simulink model "CRCL"  (R2020b)
settings: Solver=FixedStepDiscrete  StartTime=0.0  StopTime=inf  FixedStep=0.01  RelTol=1e-3  EnableMultiTasking=on
values from neighbouring files (symbols this model uses):
  calibrationDelayTime_s = 2.0    [CRCL_Dictionary.sldd]
  collisionAngleThreshold_deg = 40.0    [CRCL_Dictionary.sldd]
  collisionVarianceThreshold_g2 = 8.0    [CRCL_Dictionary.sldd]
  cpMaxAbortTime_s = 30.0    [CRCL_Dictionary.sldd]
  cpMaxTipOverAngle_deg = 35.0    [CRCL_Dictionary.sldd]
  cpMinEstDistance_m = 50.0    [CRCL_Dictionary.sldd]
  cpMinEstDistanceGnssBased_m = 200.0    [CRCL_Dictionary.sldd]
  cpMinRiddenTime_s = 15.0    [CRCL_Dictionary.sldd]
  cpMinSpeedRiding_kmh = 10.0    [CRCL_Dictionary.sldd]
  cpNumCrankRevolutionThreshold = 5.0    [CRCL_Dictionary.sldd]
  cpSpeedCond2PositiveSpeedChangeTime_s = 5.0    [CRCL_Dictionary.sldd]
  cpSpeedDerivativeThreshold_kmhs = 0.005    [CRCL_Dictionary.sldd]
  cpTimeOutSpeedCond2_s = 15.0    [CRCL_Dictionary.sldd]
  groundHitEnergyThresholdStanding_g2s2 = 0.02    [CRCL_Dictionary.sldd]
  groundHitTipOverAngleThreshold_deg = 40.0    [CRCL_Dictionary.sldd]
  longAccCompForEulerEstFlag = 0.0    [CRCL_Dictionary.sldd]
  minEnergyStrongHit_g2s2 = 0.1    [CRCL_Dictionary.sldd]
  noMotionAccVarianceThresholdSD_g2 = 0.001    [CRCL_Dictionary.sldd]
  ride1minSpeedSlow_kmh = 4.0    [CRCL_Dictionary.sldd]
  ride2minSpeed_kmh = 8.0    [CRCL_Dictionary.sldd]
  rroMaxSpeed_kmh = 5.0    [CRCL_Dictionary.sldd]
  rroMinGyrX_degs = 20.0    [CRCL_Dictionary.sldd]
  rroMonotonyThreshold_degs = -1.0    [CRCL_Dictionary.sldd]
  rroRollIntegrationAngleThreshold_degs = 20.0    [CRCL_Dictionary.sldd]
  rroUniContinuityThreshold_degs = 15.0    [CRCL_Dictionary.sldd]
  scaleFactorVarianceStrongHit = 2.0    [CRCL_Dictionary.sldd]
  sdoMaxAccVarFreeFall_g2 = 0.06    [CRCL_Dictionary.sldd]
  sdoMaxTipOverAngle_deg = 20.0    [CRCL_Dictionary.sldd]
  sdoMinAccVar_g2 = 8.0    [CRCL_Dictionary.sldd]
  sdoMinGyrXYNorm_degs = 720.0    [CRCL_Dictionary.sldd]
  sdoMinGyrXYNormFreeFall_degs = 100.0    [CRCL_Dictionary.sldd]
  sdoMinOrientationChange_deg = 120.0    [CRCL_Dictionary.sldd]
  sdoScaleFactorOrientationChange = 3.0    [CRCL_Dictionary.sldd]
  stepTime_s = 0.01    [CRCL_Dictionary.sldd]
  strongHitSafetyFactor = 2.5    [CRCL_Dictionary.sldd]
  tipOverAccZFiltTreshold_g = 0.7    [CRCL_Dictionary.sldd]
  tipOverAngleThreshold_deg = 50.0    [CRCL_Dictionary.sldd]
  tipOverMinAccZFiltNoseOver_g = 0.3    [CRCL_Dictionary.sldd]
  tipOverRollPitchRelationNoseOver = 1.5    [CRCL_Dictionary.sldd]
undefined symbols (not defined in the file or in its folder): magnitude
libraries: simulink x17
(part 6 of 8)

== matlab function CRCL/MATLAB Function1 ==
  data: probRide1 input; p_noCrash output; probRide2 input; probSoftColl input; probColl input; probStrongColl input; probTipOver input; probNoseOver input; probGroundHit input; probRRO input; probSDO input; probHubConnection input; systemConfig input; p_crash output; crashClass output; outputCrashClass output; p_maxCrashClass output; tipOverAngleFused_deg input; outputGeneralCrashClass output; p_generalCrashClass output; cobiHubSetup input; p_cc1x output; p_cc3x output; secondCalibDoneDelayed input
function [p_noCrash, p_crash, crashClass, outputCrashClass, ...
    p_maxCrashClass, outputGeneralCrashClass, ...
    p_generalCrashClass, p_cc1x, p_cc3x] = crashProbabilityFusion(probRide1, probRide2, probSoftColl, ...
    probColl, probStrongColl, probTipOver, probNoseOver, probGroundHit, ...
    probRRO, probSDO, probHubConnection, systemConfig, ...
    tipOverAngleFused_deg, cobiHubSetup, secondCalibDoneDelayed)

persistent lastCrashClass probRide1Freeze ...
    probRide2Freeze rideFeatureFreeze lastCrashClassRanking ...
    crashClassHighestRanking generalCrashClassHighestRanking ...
    generalCrashClassProb

if isempty(lastCrashClass)
    lastCrashClass = single(0);
    probRide1Freeze = single(0);
    probRide2Freeze = single(0);
    rideFeatureFreeze = int16(0);
    lastCrashClassRanking = single(0);
    crashClassHighestRanking = int16(0);
    generalCrashClassHighestRanking = int16(0);
    generalCrashClassProb = single(0);
end

%ride feature freeze 
if (tipOverAngleFused_deg >= 50 || probGroundHit >= 0.5 || ...
        probColl >= 0.5) && rideFeatureFreeze == 0 && secondCalibDoneDelayed == 1
    probRide1Freeze = probRide1;
    probRide2Freeze = probRide2;
    rideFeatureFreeze = int16(1);
%reset frozen feature states and crash classes + probs
elseif  tipOverAngleFused_deg < 50 && probGroundHit < 0.5 && ...
        probColl < 0.5 && probTipOver < 0.5 && probSDO < 0.5 && ...
        ~(probHubConnection < 0.5 && systemConfig == 2) && rideFeatureFreeze == 1
    probRide1Freeze = probRide1;
    probRide2Freeze = probRide2;
    rideFeatureFreeze = int16(0);
    lastCrashClassRanking = single(0);
    crashClassHighestRanking = int16(0);
    generalCrashClassHighestRanking = int16(0);
    generalCrashClassProb = single(0);
elseif rideFeatureFreeze == 0
     probRide1Freeze = probRide1;
     probRide2Freeze = probRide2;
end
    
%% probabilistic tree

%% ride0
if probRide1Freeze < 0.3
    p_0 = 1 - probRide1Freeze;

    %collision node
    p_00 = p_0 * (1 - probSoftColl);                                    % -> no Collision
    p_01 = p_0 * probSoftColl * (1 - probColl) ;                        % -> soft Collsion
    p_02 = p_0 * probSoftColl * probColl * (1 - probStrongColl);        % -> Collision
    p_03 = p_0 * probSoftColl * probColl * probStrongColl;              % -> Strong Collision

    % tipover
    p_000 = p_00 * (1 - probTipOver);                                   %no TipOver
    p_001 = p_00 * probTipOver * (1 - probNoseOver);                    %RollOver
    p_002 = p_00 * probTipOver * probNoseOver;                          %NoseOver

    p_010 = p_01 * (1 - probTipOver);
    p_011 = p_01 * probTipOver * (1 - probNoseOver);
    p_012 = p_01 * probTipOver * probNoseOver;

    p_020 = p_02 * (1 - probTipOver);
    p_021 = p_02 * probTipOver * (1 - probNoseOver);
    p_022 = p_02 * probTipOver * probNoseOver;

    p_030 = p_03 * (1 - probTipOver);
    p_031 = p_03 * probTipOver * (1 - probNoseOver);
    p_032 = p_03 * probTipOver * probNoseOver;

    % ground hit node
    %not riding, no Collision
    p_0000 = p_000 * (1-probGroundHit);
    p_0001 = p_000 * probGroundHit;

    p_0010 = p_001 * (1-probGroundHit);
    p_0011 = p_001 * probGroundHit;

    p_0020 = p_002 * (1-probGroundHit);
    p_0021 = p_002 * probGroundHit;

    %not riding, softCollision
    p_0100 = p_010 * (1-probGroundHit);
    p_0101 = p_010 * probGroundHit;

    p_0110 = p_011 * (1-probGroundHit);
    p_0111 = p_011 * probGroundHit;

    p_0120 = p_012 * (1-probGroundHit);
    p_0121 = p_012 * probGroundHit;

    %not riding, Collision
    p_0200 = p_020 * (1-probGroundHit);
    p_0201 = p_020 * probGroundHit;

    p_0210 = p_021 * (1-probGroundHit);
    p_0211 = p_021 * probGroundHit;

    p_0220 = p_022 * (1-probGroundHit);
    p_0221 = p_022 * probGroundHit;

    %not riding, strong Collision
    p_0300 = p_030 * (1-probGroundHit);
    p_0301 = p_030 * probGroundHit;

    p_0310 = p_031 * (1-probGroundHit);
    p_0311 = p_031 * probGroundHit;

    p_0320 = p_032 * (1-probGroundHit);
    p_0321 = p_032 * probGroundHit;

    % special features
    % riderlessRollOver
    p_0011a = p_0011 * (1 - single(probRRO));
    p_0011b = p_0011 * single(probRRO);


    p_1000 = single(0);
    p_1001 = single(0);
    p_1010 = single(0);
    p_1011 = single(0);
    p_1020 = single(0);
    p_1021 = single(0);
    p_1200 = single(0);
    p_1201 = single(0);
    p_1210 = single(0);
    p_1211 = single(0);
    p_1220 = single(0);
    p_1221 = single(0);
    p_1300 = single(0);
    p_1301 = single(0);
    p_1310 = single(0);
    p_1311 = single(0);
    p_1320 = single(0);
    p_1321 = single(0);
    
    p_2000 = single(0);
    p_2001 = single(0);
    p_2010 = single(0);
    p_2011 = single(0);
    p_2020 = single(0);
    p_2021 = single(0);
    p_2200 = single(0);
    p_2201 = single(0);
    p_2210 = single(0);
    p_2211 = single(0);
    p_2220 = single(0);
    p_2221 = single(0);
    p_2300 = single(0);
    p_2301 = single(0);
    p_2310 = single(0);
    p_2311 = single(0);
    p_2320 = single(0);
    p_2321 = single(0);

else
    %% ride1
    p_1 = probRide1Freeze * (1-probRide2Freeze);

    %collision node
    p_10 = p_1 * (1 - probColl);                                        % -> no Collison
    p_12 = p_1 * probColl * (1 - probStrongColl);                       % -> Collision
    p_13 = p_1 * probColl * probStrongColl;                             % -> strongCollsion

    % tipover
    p_100 = p_10 * (1 - probTipOver);
    p_101 = p_10 * probTipOver * (1 - probNoseOver);
    p_102 = p_10 * probTipOver * probNoseOver;

    p_120 = p_12 * (1 - probTipOver);
    p_121 = p_12 * probTipOver * (1 - probNoseOver);
    p_122 = p_12 * probTipOver * probNoseOver;

    p_130 = p_13 * (1 - probTipOver);
    p_131 = p_13 * probTipOver * (1 - probNoseOver);
    p_132 = p_13 * probTipOver * probNoseOver;

    % ground hit node
    %riding 1, no Collision
    p_1000 = p_100 * (1-probGroundHit);
    p_1001 = p_100 * probGroundHit;

    p_1010 = p_101 * (1-probGroundHit);
    p_1011 = p_101 * probGroundHit;

    p_1020 = p_102 * (1-probGroundHit);
    p_1021 = p_102 * probGroundHit;

    %riding 1, Collision
    p_1200 = p_120 * (1-probGroundHit);
    p_1201 = p_120 * probGroundHit;

    p_1210 = p_121 * (1-probGroundHit);
    p_1211 = p_121 * probGroundHit;

    p_1220 = p_122 * (1-probGroundHit);
    p_1221 = p_122 * probGroundHit;

    %riding 1, strong Collision
    p_1300 = p_130 * (1-probGroundHit);
    p_1301 = p_130 * probGroundHit;

    p_1310 = p_131 * (1-probGroundHit);
    p_1311 = p_131 * probGroundHit;

    p_1320 = p_132 * (1-probGroundHit);
    p_1321 = p_132 * probGroundHit;

    %% ride2
    p_2 = probRide1Freeze * probRide2Freeze;

    %collision node
    p_20 = p_2 * (1 - probColl);                                        % -> no Collison
    p_22 = p_2 * probColl * (1 - probStrongColl);                       % -> Collision
    p_23 = p_2 * probColl * probStrongColl;                             % -> strongCollsion

    % tipover
    p_200 = p_20 * (1 - probTipOver);
    p_201 = p_20 * probTipOver * (1 - probNoseOver);
    p_202 = p_20 * probTipOver * probNoseOver;

    p_220 = p_22 * (1 - probTipOver);
    p_221 = p_22 * probTipOver * (1 - probNoseOver);
    p_222 = p_22 * probTipOver * probNoseOver;

    p_230 = p_23 * (1 - probTipOver);
    p_231 = p_23 * probTipOver * (1 - probNoseOver);
    p_232 = p_23 * probTipOver * probNoseOver;

    % ground hit node
    %riding 2, no Collision
    p_2000 = p_200 * (1-probGroundHit);
    p_2001 = p_200 * probGroundHit;

    p_2010 = p_201 * (1-probGroundHit);
    p_2011 = p_201 * probGroundHit;

    p_2020 = p_202 * (1-probGroundHit);
    p_2021 = p_202 * probGroundHit;

    %riding 2, Collision
    p_2200 = p_220 * (1-probGroundHit);
    p_2201 = p_220 * probGroundHit;

    p_2210 = p_221 * (1-probGroundHit);
    p_2211 = p_221 * probGroundHit;

    p_2220 = p_222 * (1-probGroundHit);
    p_2221 = p_222 * probGroundHit;

    %riding 2, strong Collision
    p_2300 = p_230 * (1-probGroundHit);
    p_2301 = p_230 * probGroundHit;

    p_2310 = p_231 * (1-probGroundHit);
    p_2311 = p_231 * probGroundHit;

    p_2320 = p_232 * (1-probGroundHit);
    p_2321 = p_232 * probGroundHit;
    
    p_0000 = single(0);
    p_0001 = single(0);
    p_0010 = single(0);
    %p_0011 = single(0);
    p_0020 = single(0);
    p_0021 = single(0);
    p_0100 = single(0);
    p_0101 = single(0);
    p_0110 = single(0);
    p_0111 = single(0);
    p_0120 = single(0);
    p_0121 = single(0);
    p_0200 = single(0);
    p_0201 = single(0);
    p_0210 = single(0);
    p_0211 = single(0);
    p_0220 = single(0);
    p_0221 = single(0);
    p_0300 = single(0);
    p_0301 = single(0);
    p_0310 = single(0);
    p_0311 = single(0);
    p_0320 = single(0);
    p_0321 = single(0);
    p_0011a = single(0);
    p_0011b = single(0);
end

%% crashClasses

%no crash
p_cc00 = p_0000 + p_0001 + p_0010 + p_0020 + p_0100 + p_0101 + p_0110 + ...
    p_0120 + p_0200 + p_0201 + p_1000 + p_1001 + p_1010 + p_1020 + ...
    p_1200 + p_1201 + p_2000 + p_2001 + p_2200 + p_2201;
p_cc70 = p_0011b;
p_maxCrashClass = p_cc00;

crashClass = int16(0);
if lastCrashClassRanking <= 5 && p_cc00 > 0.5
    lastCrashClassRanking = single(5);
    crashClassHighestRanking = crashClass;
    generalCrashClassHighestRanking = int16(0);
    generalCrashClassProb = p_cc00 + p_cc70;
end


if p_cc70 > p_maxCrashClass
    p_maxCrashClass = p_cc70;
    crashClass = int16(70);
    if lastCrashClassRanking <= 7 && p_cc70 > 0.5
        lastCrashClassRanking = single(7);
        crashClassHighestRanking = crashClass;
        generalCrashClassHighestRanking = int16(0);
        generalCrashClassProb = p_cc00 + p_cc70;
    end
end

% crashes
p_cc10 = p_1210 + p_1211 + p_2210 + p_2211;
p_cc11 = p_1300 + p_1301 + p_2300 + p_2301;
p_cc12 = p_1220 + p_1221 + p_2220 + p_2221;
p_cc15 = p_1310 + p_1311 + p_2310 + p_2311;
p_cc16 = p_1320 + p_1321 + p_2320 + p_2321;

p_cc1x = p_cc10 + p_cc11 + p_cc12 + p_cc15 + p_cc16;

if p_cc10 > p_maxCrashClass
    p_maxCrashClass = p_cc10;
    crashClass = int16(10);
    if lastCrashClassRanking <= 30 && p_cc10 > 0.5
        lastCrashClassRanking = single(30);
        crashClassHighestRanking = crashClass;
        generalCrashClassHighestRanking = int16(1);
        generalCrashClassProb = p_cc1x;
    end
end
if p_cc11 > p_maxCrashClass
    p_maxCrashClass = p_cc11;
    crashClass = int16(11);
    if lastCrashClassRanking <= 25 && p_cc11 > 0.5
        lastCrashClassRanking = single(25);
        crashClassHighestRanking = crashClass;
        generalCrashClassHighestRanking = int16(1);
        generalCrashClassProb = p_cc1x;
    end
end
if p_cc12 > p_maxCrashClass
    p_maxCrashClass = p_cc12;
    crashClass = int16(12);
    if lastCrashClassRanking <= 30 && p_cc12 > 0.5
        lastCrashClassRanking = single(30);
        crashClassHighestRanking = crashClass;
        generalCrashClassHighestRanking = int16(1);
        generalCrashClassProb = p_cc1x;
    end
end
if p_cc15 > p_maxCrashClass
    p_maxCrashClass = p_cc15;
    crashClass = int16(15);
    if lastCrashClassRanking <= 30 && p_cc15 > 0.5
        lastCrashClassRanking = single(30);
        crashClassHighestRanking = crashClass;
        generalCrashClassHighestRanking = int16(1);
        generalCrashClassProb = p_cc1x;
    end
end
if p_cc16 > p_maxCrashClass
    p_maxCrashClass = p_cc16;
    crashClass = int16(16);
    if lastCrashClassRanking <= 30 && p_cc16 > 0.5
        lastCrashClassRanking = single(30);
        crashClassHighestRanking = crashClass;
        generalCrashClassHighestRanking = int16(1);
        generalCrashClassProb = p_cc1x;
    end
end

p_cc20 = p_2010 + p_2011;
p_cc22 = p_2020 + p_2021;

p_cc2x = p_cc20 + p_cc22;

if p_cc20 > p_maxCrashClass
    p_maxCrashClass = p_cc20;
    crashClass = int16(20);
    if lastCrashClassRanking <= 20 && p_cc20 > 0.5
        lastCrashClassRanking = single(20);
        crashClassHighestRanking = crashClass;
        generalCrashClassHighestRanking = int16(2);
        generalCrashClassProb = p_cc2x;
    end
end
if p_cc22 > p_maxCrashClass
    p_maxCrashClass = p_cc22;
    crashClass = int16(22);
    if lastCrashClassRanking <= 20 && p_cc22 > 0.5
        lastCrashClassRanking = single(20);
        crashClassHighestRanking = crashClass;
        generalCrashClassHighestRanking = int16(2);
        generalCrashClassProb = p_cc2x;
    end
end

p_cc30 = p_1011;
p_cc32 = p_1021;
p_cc33 = p_0011a + p_0021;

p_cc3x = p_cc30 + p_cc32 + p_cc33;

if p_cc30 > p_maxCrashClass 
    p_maxCrashClass = p_cc30;
    crashClass = int16(30);
    if lastCrashClassRanking <= 25 && p_cc30 > 0.5
        lastCrashClassRanking = single(25);
        crashClassHighestRanking = crashClass;
        generalCrashClassHighestRanking = int16(3);
        generalCrashClassProb = p_cc3x;
    end
end
if p_cc32 > p_maxCrashClass
    p_maxCrashClass = p_cc32;
    crashClass = int16(32);
    if lastCrashClassRanking <= 25 && p_cc32 > 0.5
        lastCrashClassRanking = single(25);
        crashClassHighestRanking = crashClass;
        generalCrashClassHighestRanking = int16(3);
        generalCrashClassProb = p_cc3x;
    end
end
if p_cc33 > p_maxCrashClass
    p_maxCrashClass = p_cc33;
    crashClass = int16(33);
    if lastCrashClassRanking <= 15 && p_cc33 > 0.5
        lastCrashClassRanking = single(15);
        crashClassHighestRanking = crashClass;
        generalCrashClassHighestRanking = int16(3);
        generalCrashClassProb = p_cc3x;
    end
end


p_cc40 = p_0111 + p_0121;
p_cc41 = p_0300 + p_0301;
p_cc44 = p_0210 + p_0211 + p_0220 + p_0221;
p_cc45 = p_0310 + p_0311 + p_0320 + p_0321;
p_cc4x = p_cc41 + p_cc40 + p_cc44 + p_cc45;

if p_cc40 > p_maxCrashClass
    p_maxCrashClass = p_cc40;
    crashClass = int16(40);
    if lastCrashClassRanking <= 25 && p_cc40 > 0.5
        lastCrashClassRanking = single(25);
        crashClassHighestRanking = crashClass;
        generalCrashClassHighestRanking = int16(4);
        generalCrashClassProb = p_cc4x;
    end
end
if p_cc41 > p_maxCrashClass
    p_maxCrashClass = p_cc41;
    crashClass = int16(41);
    if lastCrashClassRanking <= 10 && p_cc41 > 0.5
        lastCrashClassRanking = single(10);
        crashClassHighestRanking = crashClass;
        generalCrashClassHighestRanking = int16(4);
        generalCrashClassProb = p_cc4x;
    end
end
if p_cc44 > p_maxCrashClass
    p_maxCrashClass = p_cc44;
    crashClass = int16(44);
    if lastCrashClassRanking <= 20 && p_cc44 > 0.5
        lastCrashClassRanking = single(20);
        crashClassHighestRanking = crashClass;
        generalCrashClassHighestRanking = int16(4);
        generalCrashClassProb = p_cc4x;
    end
end
if p_cc45 > p_maxCrashClass
    p_maxCrashClass = p_cc45;
    crashClass = int16(45);
    if lastCrashClassRanking <= 20 && p_cc45 > 0.5
        lastCrashClassRanking = single(20);
        crashClassHighestRanking = crashClass;
        generalCrashClassHighestRanking = int16(4);
        generalCrashClassProb = p_cc4x;
    end
end




%% output 
p_noCrash = p_cc00 + p_cc70;

p_crash = p_cc10 + p_cc11 + p_cc12 + p_cc15 + p_cc16 + p_cc20 + p_cc22 + ...
    p_cc30 + p_cc32 + p_cc33 + p_cc40 + p_cc41 + p_cc44 + p_cc45;

% cobi special cases
if systemConfig == 2 && probHubConnection == 0  && ... % lost hub
        cobiHubSetup ~= 1 && ...
        (probColl >= 0.5 || probGroundHit >= 0.5)
    lastCrashClassRanking = single(50);
    generalCrashClassHighestRanking = int16(8);
    generalCrashClassProb = single(1);
    if probRide1Freeze >= 0.5   %riding
        crashClass = int16(81);
        crashClassHighestRanking = crashClass;
        lastCrashClassRanking = single(55);
        %p_maxCrashClass = single(1);
    else                            % not riding
        crashClass = int16(80);
        crashClassHighestRanking = crashClass;
        lastCrashClassRanking = single(50);
        %p_maxCrashClass = single(1);    
    end
elseif systemConfig == 2 && probHubConnection == 1 && ...
        probSDO >= 0.9 % smartphone drop out cases
    p_crash = single(1);
    p_noCrash = single(0);
    generalCrashClassHighestRanking = int16(8);
    generalCrashClassProb = single(1);
    if lastCrashClassRanking < single(50)
        if probRide1Freeze >= 0.5   %riding
            crashClass = int16(83);
            crashClassHighestRanking = crashClass;
            lastCrashClassRanking = single(45);
            %p_maxCrashClass = single(1);
        else                        %not riding
            crashClass = int16(82);
            crashClassHighestRanking = crashClass;
            lastCrashClassRanking = single(40);
            %p_maxCrashClass = single(1);   
        end
    end
end

outputCrashClass = crashClassHighestRanking;
outputGeneralCrashClass = generalCrashClassHighestRanking;
p_generalCrashClass = generalCrashClassProb;

% if
%     outputCrashClass
% else
%     outputCrashClass
% end

end

== stateflow chart CRCL/CP_crashPlausiblizer ==
  state plausibilityChecker [parallel]
    settings: executionOrder=1
    state Idle_
      en:
      CP_fire = int16(0);
      CP_crashAborted = int16(0);
      CP_plausibleCrashClass =int16(0);
    state plausibleCrash
      en:
      CP_fire = int16(1);
      CP_plausibleCrashClass =CP_crashClassTmp;
      du:
      if CP_curCrashClass ~=0  && ...
      CP_crashClassTmp ~= CP_curCrashClass
      CP_crashClassTmp = CP_curCrashClass;
      CP_plausibleCrashClass =CP_crashClassTmp;
      end
    state CrashDetected
      du:
      if CP_curCrashClass ~=0  && ...
      CP_crashClassTmp ~= CP_curCrashClass
      CP_crashClassTmp = CP_curCrashClass;
      end
    state unplausibleCrash
      en:
      CP_crashAborted = int16(1);
    plausibleCrash -> Idle_ : [CP_crashFire == 0 && after(5,sec)]
    (default) -> Idle_
    Idle_ -> plausibilityChecker.CrashDetected : [CP_crashFire ==1]
        | {
        | CP_crashClassTmp = CP_curCrashClass;
        | }
    plausibilityChecker.CrashDetected -> plausibleCrash [order 1] : [CP_standFire || ...
        | CP_crashClass >= 80 || ...
        | CP_curSpeed_kmh < CP_minSpeedRiding_kmh || ...
        | after(CP_maxAbortTime_s,sec)]
        | %&& ...
        | %CP_speedCondFire == 0 && ...
        | %CP_cadenceCondFire == 0 && ...
        | %CP_speedCond2Fire == 0)]
    plausibilityChecker.CrashDetected -> unplausibleCrash [order 2] : [CP_speedCondFire == 2 || ...
        | CP_cadenceCondFire == 2 || ...
        | CP_speedCond2Fire == 2 || ...
        | CP_gnssSpeedCondFire == 2]
    unplausibleCrash -> Idle_ : [CP_crashFire == 0]
  state speedUprigthBikeConditionChecker [parallel]
    settings: executionOrder=2
    state waitState
    state SpeedConditionValid
      en:
      CP_speedCondFire = int16(1);
      CP_intDistance_m = CP_timeStep_s * CP_curSpeed_kmh/3.6;
      du:
      CP_intDistance_m  = CP_intDistance_m + CP_timeStep_s * CP_curSpeed_kmh/3.6;
    state Idle
      en:
      CP_speedCondFire = int16(0);
    state CrashDetected
      en:
      CP_speedCondFire = int16(0);
    state wait
    speedUprigthBikeConditionChecker.SpeedConditionValid -> speedUprigthBikeConditionChecker.waitState [order 1] : [after(CP_minRiddenTime_s,sec) && CP_intDistance_m >= CP_minEstDistance_m]
        | {
        | CP_speedCondFire = int16(2);
        | }
    speedUprigthBikeConditionChecker.waitState -> speedUprigthBikeConditionChecker.Idle : [after(1,sec)]
    speedUprigthBikeConditionChecker.Idle -> speedUprigthBikeConditionChecker.CrashDetected [commented out] : [CP_crashFire ==1]
    speedUprigthBikeConditionChecker.CrashDetected -> speedUprigthBikeConditionChecker.SpeedConditionValid [order 1] : %check if bicycle is upright and backwheel is rotating
        | [CP_curSpeed_kmh > CP_minSpeedRiding_kmh && ...
        | (CP_tipOverAngleFused_deg <= CP_maxTipOverAngle_deg && ...
        | CP_tipOverAngleAcc_deg <= CP_maxTipOverAngle_deg)]
    speedUprigthBikeConditionChecker.CrashDetected -> speedUprigthBikeConditionChecker.Idle [commented out] : [CP_crashFire ==0 && after(15,sec)]
    (default) -> speedUprigthBikeConditionChecker.Idle
    speedUprigthBikeConditionChecker.SpeedConditionValid -> speedUprigthBikeConditionChecker.CrashDetected [order 2] : [CP_curSpeed_kmh < CP_minSpeedRiding_kmh || ...
        | CP_tipOverAngleFused_deg > CP_maxTipOverAngle_deg || ...
        | CP_tipOverAngleAcc_deg > CP_maxTipOverAngle_deg]
    speedUprigthBikeConditionChecker.Idle -> speedUprigthBikeConditionChecker.CrashDetected [order 1] : [CP_crashFire ==1 && ...
        | CP_curSpeed_kmh >= CP_minSpeedRiding_kmh]
    speedUprigthBikeConditionChecker.CrashDetected -> speedUprigthBikeConditionChecker.wait [order 2] : [CP_curSpeed_kmh < CP_minSpeedRiding_kmh || after(CP_maxAbortTime_s,sec)]
    speedUprigthBikeConditionChecker.wait -> speedUprigthBikeConditionChecker.Idle : [CP_crashFire ==0]
    speedUprigthBikeConditionChecker.Idle -> speedUprigthBikeConditionChecker.wait [order 2] : [CP_crashFire ==1 && ...
        | CP_curSpeed_kmh < CP_minSpeedRiding_kmh]
  state cadenceConditionChecker [parallel]
    settings: executionOrder=3
    state waitState
    state Idle
      en:
      CP_cadenceCondFire = int16(0);
    state checkCadenceCondition
      en:
      CP_cadenceCondFire = int16(1);
      du:
      CP_crankRotation = CP_curCadence/60 * CP_timeStep_s + CP_crankRotation;
    state CrashDetected
      en:
      CP_cadenceCondFire = int16(0);
      CP_crankRotation = single(0);
    state waitState1
    state wait
      en:
      CP_cadenceCondFire = int16(0);
    cadenceConditionChecker.waitState -> cadenceConditionChecker.Idle : [after(1,sec)]
    checkCadenceCondition -> cadenceConditionChecker.waitState [order 2] : %cadence condition valid
        | [CP_crankRotation >= CP_numCrankRevolutionThreshold]
        | {
        | CP_cadenceCondFire = int16(2);
        | }
    cadenceConditionChecker.CrashDetected -> checkCadenceCondition [order 1] : %check if user applies valid cadence
        | [CP_curCadence >= 30 && CP_curCadence <= 150]
        | %(CP_tipOverAngleFused_deg <= 35 && ...
        | %CP_tipOverAngleAcc_deg <= 35)]
    cadenceConditionChecker.Idle -> cadenceConditionChecker.CrashDetected [order 1] : [CP_crashFire ==1 && ...
        | CP_curSpeed_kmh > CP_minSpeedRiding_kmh]
    (default) -> cadenceConditionChecker.Idle
    checkCadenceCondition -> waitState1 [order 1] : [CP_curCadence < 30 || ...
        | CP_curCadence > 150]
    cadenceConditionChecker.CrashDetected -> cadenceConditionChecker.Idle [commented out] : [CP_crashFire == 0 && after(25,sec)]
    waitState1 -> cadenceConditionChecker.CrashDetected [order 2] : [after(5,sec)]
    waitState1 -> checkCadenceCondition [order 1] : [CP_curCadence >= 30  && ...
        | CP_curCadence <= 150]
    cadenceConditionChecker.CrashDetected -> cadenceConditionChecker.wait [order 2] : [CP_curSpeed_kmh < CP_minSpeedRiding_kmh || ...
        |  after(CP_maxAbortTime_s,sec)]
    waitState1 -> cadenceConditionChecker.wait [order 3] : [CP_curSpeed_kmh < CP_minSpeedRiding_kmh]
    cadenceConditionChecker.wait -> cadenceConditionChecker.Idle : [CP_crashFire ==0]
    cadenceConditionChecker.Idle -> cadenceConditionChecker.wait [order 2] : [CP_crashFire ==1 && ...
        | CP_curSpeed_kmh < CP_minSpeedRiding_kmh]
  state speedCondition2Checker [parallel]
    settings: executionOrder=4
    state CheckSpeedDerivative4
      en:
    state waitState
    state CheckPositiveSpeedDerivative2
      en:
    note: check if speed signal is not showing off the characteristics
        | of a rolling out back wheel (after a rollOver)
        | even if the estimated orientation of the bicycle looks like some sort of tipOver (Liuba Case)
    state CheckSpeedDerivative3
      en:
    state Idle
      en:
      CP_speedCond2Fire = int16(0);
    state CrashDetected
      en:
      %CP_speedCond2Fire = int16(0);
    state CheckSpeedDerivative
      en:
    state wait
      en:
      CP_speedCond2Fire = int16(0);
    state CheckPositiveSpeedDerivative1
      en:
    state CheckPositiveSpeedDerivative [commented out]
      en:
    state CheckSpeedDerivative1
      en:
    state CheckSpeedDerivative2
      en:
    CheckPositiveSpeedDerivative2 -> CheckSpeedDerivative4 [order 1] : [CP_curSpeedDerivative < 0]
    CheckPositiveSpeedDerivative2 -> speedCondition2Checker.waitState [order 2] : [after(CP_speedCond2PositiveSpeedChangeTime_s,sec)]
        | {
        | CP_speedCond2Fire = int16(2);
        | }
    CheckSpeedDerivative4 -> CheckPositiveSpeedDerivative2 [order 3] : [CP_curSpeedDerivative >= 0 &&...
        | CP_curSpeed_kmh > CP_minSpeedRiding_kmh]
    CheckSpeedDerivative4 -> speedCondition2Checker.waitState [order 1] : [CP_curSpeedDerivative < -CP_speedDerivativeThreshold_kmhs &&...
        | CP_curSpeed_kmh > CP_minSpeedRiding_kmh]
        | {
        | CP_speedCond2Fire = int16(2);
        | }
    speedCondition2Checker.waitState -> speedCondition2Checker.Idle : [after(1,sec)]
    CheckSpeedDerivative4 -> (junction 89) [order 2] : [(CP_crashFire == 0 && ...
        |  after(CP_timeOutSpeedCond2_s,sec)) || ...
        | CP_curSpeed_kmh < CP_minSpeedRiding_kmh]
    CheckSpeedDerivative3 -> CheckSpeedDerivative4 [order 1] : [CP_curSpeedDerivative > CP_speedDerivativeThreshold_kmhs &&...
        | CP_curSpeed_kmh > CP_minSpeedRiding_kmh]
    speedCondition2Checker.Idle -> speedCondition2Checker.CrashDetected [order 1] : [CP_crashFire ==1 && CP_curSpeed_kmh > CP_minSpeedRiding_kmh]
    speedCondition2Checker.CrashDetected -> CheckSpeedDerivative [order 1] : [CP_curSpeedDerivative > ...
        | CP_speedDerivativeThreshold_kmhs &&...
        | CP_curSpeed_kmh > CP_minSpeedRiding_kmh]
    (default) -> speedCondition2Checker.Idle
    speedCondition2Checker.CrashDetected -> speedCondition2Checker.Idle [commented out] : [CP_crashFire ==0 && after(CP_timeOutSpeedCond2,sec)]
    speedCondition2Checker.CrashDetected -> speedCondition2Checker.Idle [commented out] : [CP_crashFire ==0 && CP_curSpeed_kmh < CP_minSpeedRiding_kmh]
    CheckSpeedDerivative3 -> (junction 89) [order 2] : [(CP_crashFire == 0 && ...
        |  after(CP_timeOutSpeedCond2_s,sec)) || ...
        | CP_curSpeed_kmh < CP_minSpeedRiding_kmh]
    CheckSpeedDerivative2 -> CheckSpeedDerivative3 [order 1] : [CP_curSpeedDerivative < -CP_speedDerivativeThreshold_kmhs &&...
        | CP_curSpeed_kmh > CP_minSpeedRiding_kmh]
    CheckPositiveSpeedDerivative1 -> CheckSpeedDerivative3 [order 2] : [after(CP_speedCond2PositiveSpeedChangeTime_s,sec)]
    CheckSpeedDerivative -> CheckPositiveSpeedDerivative [commented out] : [CP_curSpeedDerivative >= 0 &&...
        | CP_curSpeed_kmh > CP_minSpeedRiding_kmh]
    CheckPositiveSpeedDerivative -> CheckSpeedDerivative [commented out] : [CP_curSpeedDerivative < 0]
    CheckSpeedDerivative -> CheckSpeedDerivative1 [order 2] : [CP_curSpeedDerivative < -CP_speedDerivativeThreshold_kmhs &&...
        | CP_curSpeed_kmh > CP_minSpeedRiding_kmh]
    CheckSpeedDerivative -> (junction 89) [order 1] : [(CP_crashFire == 0 && ...
        |  after(CP_timeOutSpeedCond2_s,sec)) || ...
        | CP_curSpeed_kmh < CP_minSpeedRiding_kmh]
    speedCondition2Checker.CrashDetected -> speedCondition2Checker.wait [order 2] : [CP_curSpeed_kmh < CP_minSpeedRiding_kmh || after(CP_maxAbortTime_s,sec)]
    speedCondition2Checker.wait -> speedCondition2Checker.Idle : [CP_crashFire ==0]
    speedCondition2Checker.Idle -> speedCondition2Checker.wait [order 2] : [CP_crashFire ==1 && ...
        | CP_curSpeed_kmh < CP_minSpeedRiding_kmh]
    (junction 89) -> speedCondition2Checker.wait
    CheckSpeedDerivative2 -> (junction 89) [order 3] : [(CP_crashFire == 0 && ...
        |  after(CP_timeOutSpeedCond2_s,sec)) || ...
        | CP_curSpeed_kmh < CP_minSpeedRiding_kmh]
    CheckSpeedDerivative1 -> (junction 89) [order 2] : [(CP_crashFire == 0 && ...
        |  after(CP_timeOutSpeedCond2_s,sec)) || ...
        | CP_curSpeed_kmh < CP_minSpeedRiding_kmh]
    CheckSpeedDerivative2 -> CheckPositiveSpeedDerivative1 [order 2] : [CP_curSpeedDerivative >= 0 &&...
        | CP_curSpeed_kmh > CP_minSpeedRiding_kmh]
    CheckPositiveSpeedDerivative1 -> CheckSpeedDerivative2 [order 1] : [CP_curSpeedDerivative < 0]
    CheckPositiveSpeedDerivative -> CheckSpeedDerivative1 [commented out] : [after(CP_speedCond2PositiveSpeedChangeTime_s,sec)]
    CheckSpeedDerivative1 -> CheckSpeedDerivative2 [order 1] : [CP_curSpeedDerivative > CP_speedDerivativeThreshold_kmhs &&...
        | CP_curSpeed_kmh > CP_minSpeedRiding_kmh]
        | {
        | CP_speedCond2Fire = int16(1);
        | }
  state speedConditionCheckGnssBased [parallel]
    settings: executionOrder=5
    state waitState
    state SpeedConditionValid
      en:
      CP_gnssSpeedCondFire = int16(1);
      CP_intDistanceGnssBased_m = CP_timeStep_s * CP_curSpeed_kmh/3.6;
      du:
      CP_intDistanceGnssBased_m  = CP_intDistanceGnssBased_m + CP_timeStep_s * CP_curSpeed_kmh/3.6;
    state Idle
      en:
      CP_gnssSpeedCondFire = int16(0);
    state CrashDetected
      en:
      CP_gnssSpeedCondFire = int16(0);
    state wait
    speedConditionCheckGnssBased.SpeedConditionValid -> speedConditionCheckGnssBased.waitState [order 1] : [after(CP_minRiddenTime_s,sec) && ...
        | CP_intDistanceGnssBased_m >= CP_minEstDistanceGnssBased_m]
        | {
        | CP_gnssSpeedCondFire = int16(2);
        | }
    speedConditionCheckGnssBased.waitState -> speedConditionCheckGnssBased.Idle : [after(1,sec)]
    speedConditionCheckGnssBased.Idle -> speedConditionCheckGnssBased.CrashDetected [commented out] : [CP_crashFire ==1]
    speedConditionCheckGnssBased.CrashDetected -> speedConditionCheckGnssBased.SpeedConditionValid [order 1] : %check if GNSS speed is used -> hubSetup == 1!
        | [CP_curSpeed_kmh > CP_minSpeedRiding_kmh && ...
        | CP_hubSetup == 1]
    speedConditionCheckGnssBased.CrashDetected -> speedConditionCheckGnssBased.Idle [commented out] : [CP_crashFire ==0 && after(15,sec)]
    (default) -> speedConditionCheckGnssBased.Idle
    speedConditionCheckGnssBased.Idle -> speedConditionCheckGnssBased.CrashDetected [order 1] : [CP_crashFire ==1]
    speedConditionCheckGnssBased.CrashDetected -> speedConditionCheckGnssBased.wait [order 2] : [CP_curSpeed_kmh < CP_minSpeedRiding_kmh || after(CP_maxAbortTime_s,sec)]
    speedConditionCheckGnssBased.wait -> speedConditionCheckGnssBased.Idle : [CP_crashFire ==0]
    speedConditionCheckGnssBased.Idle -> speedConditionCheckGnssBased.wait [order 2] : [CP_crashFire ==1 && ...
        | CP_curSpeed_kmh < CP_minSpeedRiding_kmh]
    speedConditionCheckGnssBased.SpeedConditionValid -> speedConditionCheckGnssBased.wait [order 2] : [CP_curSpeed_kmh < CP_minSpeedRiding_kmh || after(CP_maxAbortTime_s,sec)]
  data: CP_crashFire input; CP_cadenceCondFire local; CP_standFire input; CP_curSpeed_kmh input; CP_tipOverAngleAcc_deg input; CP_tipOverAngleFused_deg input; CP_crashAborted output; CP_fire output; CP_speedCondFire local; CP_crashClass input; CP_curCadence input; CP_timeStep_s input; CP_crankRotation local; CP_curSpeedDerivative input; CP_speedCond2Fire local; CP_curCrashClass input; CP_plausibleCrashClass output; CP_crashClassTmp local; CP_intDistance_m output; CP_maxAbortTime_s input; CP_minSpeedRiding_kmh input; CP_numCrankRevolutionThreshold input; CP_minEstDistance_m input; CP_minRiddenTime_s input; CP_timeOutSpeedCond2_s input; CP_speedCond2PositiveSpeedChangeTime_s input; CP_speedDerivativeThreshold_kmhs input; CP_maxTipOverAngle_deg input; CP_gnssSpeedCondFire local; CP_hubSetup input; CP_minEstDistanceGnssBased_m input; CP_intDistanceGnssBased_m output

== stateflow chart CRCL/risingEdgeTrigger_RET ==
  state Init
    en:
    RET_lastValue = int16(0);
    RET_OutDelayed = int16(0);
  state Idle
  state waitState
    en:
    RET_output = int16(1);
  state End
    during:
    RET_lastValue = RET_curValue;
  (default) -> Init
  Init -> Idle
  End -> waitState : %reinitialize euler estimation
      | [RET_curValue == 2 && RET_lastValue == 1]
  Idle -> waitState [order 1] : [RET_lastValue == 0 && RET_curValue >= 1]
  Idle -> (junction 6) [order 2] : {
      | RET_output = int16(0);
      | }
  (junction 6) -> Idle : {
      | RET_lastValue = RET_curValue;
      | }
  waitState -> End : [after(RET_Latchtime,sec)]
      | {
      | RET_output = int16(0);
      | RET_OutDelayed = int16(1);
      | }
  data: RET_curValue input; RET_output output; RET_lastValue local; RET_OutDelayed output; RET_Latchtime input
